simulink library "Actuators"  (R2023a)
settings: Solver=VariableStepAuto  StartTime=0.0  StopTime=10.0  RelTol=1e-3
settings Model: Creator=igmso  LastModifiedBy=igmso

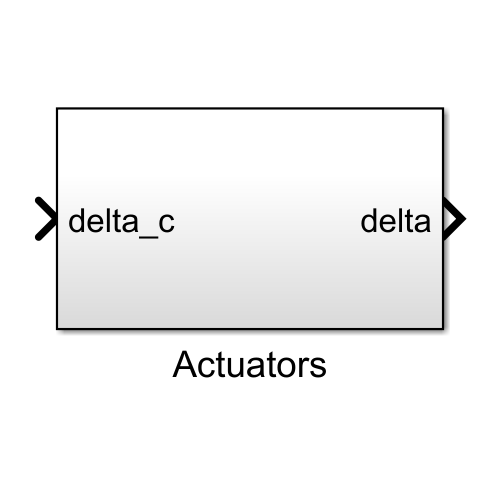
[thumbnail: Simulink's stored preview of the top-level diagram]
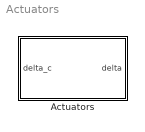
== system Actuators ==
  Actuators : Subsystem

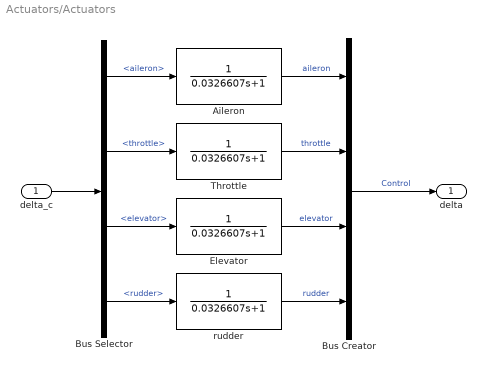
== system Actuators/Actuators ==
  delta_c : Inport
  Aileron : TransferFcn  Numerator=[0 1]  Denominator=[0.0326607 1]
  Bus Selector : BusSelector  OutputSignals=aileron,throttle,elevator,rudder
  Bus Creator : BusCreator  Inputs=4
  Elevator : TransferFcn  Numerator=[0 1]  Denominator=[0.0326607 1]
  Throttle : TransferFcn  Numerator=[0 1]  Denominator=[0.0326607 1]
  rudder : TransferFcn  Numerator=[0 1]  Denominator=[0.0326607 1]
  delta : Outport
  wires:
  delta_c/1 -> Bus Selector/1
  Bus Creator/1 -> delta/1  "Control"
  Bus Selector/1 -> Aileron/1  "<aileron>"
  Bus Selector/2 -> Throttle/1  "<throttle>"
  Bus Selector/3 -> Elevator/1  "<elevator>"
  Bus Selector/4 -> rudder/1  "<rudder>"
  Aileron/1 -> Bus Creator/1  "aileron"
  Throttle/1 -> Bus Creator/2  "throttle"
  Elevator/1 -> Bus Creator/3  "elevator"
  rudder/1 -> Bus Creator/4  "rudder"
